simulink model "modello_assey"  (R2021a)
settings: Solver=VariableStepAuto  StartTime=0.0  StopTime=0.2  RelTol=1e-3
InitFcn:
  | global pary;
  | 
  | pary = parametriy();
undefined symbols (not defined in the file or in its folder): accelerazioniy
settings Model: Creator=user  LastModifiedBy=stefa
settings SolverCC: AlgebraicLoopSolver=TrustRegion
settings DebuggingCC: SFMachineParentedDataDiag=warning

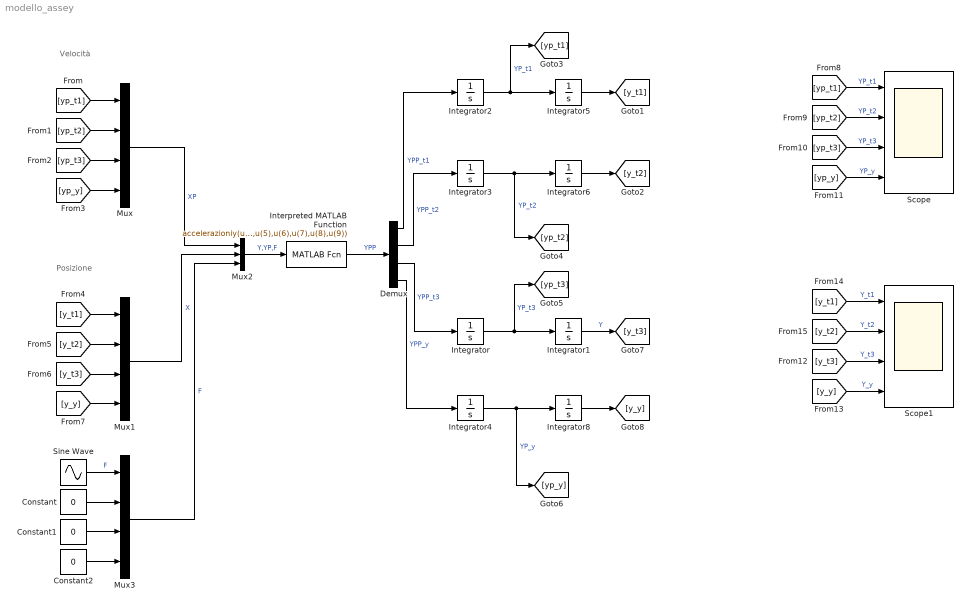
== system modello_assey ==
  note: Posizione
  note: Velocità
  Constant : Constant  Value=0
  Constant1 : Constant  Value=0
  Constant2 : Constant  Value=0
  Demux : Demux
  Integrator{,2..4} (4 alike) : Integrator
  Integrator1 : Integrator  InitialCondition=pary.Vy(3,pary.i)
  Integrator5 : Integrator  InitialCondition=pary.Vy(1,pary.i)
  Integrator6 : Integrator  InitialCondition=pary.Vy(2,pary.i)
  Integrator8 : Integrator  InitialCondition=pary.Vy(4,pary.i)
  Interpreted MATLAB Function : MATLABFcn  MATLABFcn=accelerazioniy(u(1),u(2),u(3),u(4),u(5),u(6),u(7),u(8),u(9))  OutputDimensions=4
  Mux : Mux
  Mux1 : Mux
  Mux2 : Mux  Inputs=3
  Mux3 : Mux
  Scope : Scope  NumInputPorts=4
  Scope1 : Scope  NumInputPorts=4
  Sine Wave : Sin  Amplitude=0  Frequency=200  SampleTime=0
  wires:
  [yp_t1] -> Mux/1
  [yp_t2] -> Mux/2
  [yp_t3] -> Mux/3
  [yp_y] -> Mux/4
  [y_t3] -> Mux1/3
  [y_t1] -> Mux1/1
  [y_t2] -> Mux1/2
  [y_y] -> Mux1/4
  Mux2/1 -> Interpreted MATLAB Function/1  "Y,YP,F"
  Mux/1 -> Mux2/1  "XP"
  Mux1/1 -> Mux2/2  "X"
  [yp_y] -> Scope/4  "YP_y"
  [yp_t3] -> Scope/3  "YP_t3"
  [yp_t2] -> Scope/2  "YP_t2"
  [yp_t1] -> Scope/1  "YP_t1"
  [y_t2] -> Scope1/2  "Y_t2"
  [y_t3] -> Scope1/3  "Y_t3"
  [y_y] -> Scope1/4  "Y_y"
  [y_t1] -> Scope1/1  "Y_t1"
  Demux/1 -> Integrator2/1  "YPP_t1"
  Demux/2 -> Integrator3/1  "YPP_t2"
  Demux/3 -> Integrator/1  "YPP_t3"
  Demux/4 -> Integrator4/1  "YPP_y"
  Integrator2/1 -> [yp_t1], Integrator5/1  "YP_t1"
  Integrator3/1 -> [yp_t2], Integrator6/1  "YP_t2"
  Integrator/1 -> [yp_t3], Integrator1/1  "YP_t3"
  Integrator4/1 -> [yp_y], Integrator8/1  "YP_y"
  Integrator5/1 -> [y_t1]
  Integrator6/1 -> [y_t2]
  Integrator1/1 -> [y_t3]  "Y"
  Integrator8/1 -> [y_y]
  Sine Wave/1 -> Mux3/1  "F"
  Constant/1 -> Mux3/2
  Constant1/1 -> Mux3/3
  Constant2/1 -> Mux3/4
  Mux3/1 -> Mux2/3  "F"
  Interpreted MATLAB Function/1 -> Demux/1  "YPP"
